simulink model "starship_sim"  (R2024b)
settings: Solver=VariableStepAuto  StartTime=0.0  StopTime=10  FixedStep=0.01
values from neighbouring files (symbols this model uses):
  A = [0   1   0   0   0   0    0    0    0    0 ... (first row only)    [LQR_FINAL.m]
  B = [0          0             0            0 ... (first row only)    [LQR_FINAL.m]
  C = eye(10)    [LQR_FINAL.m]
  m = 2.5    [LQR_FINAL.m]
undefined symbols (not defined in the file or in its folder): K, X, Y, Z
libraries: nesl_utility x31, sm_lib x28, sharedtransform x1
(part 1 of 2)
settings Model: Creator=gilli  LastModifiedBy=thurf
settings DebuggingCC: UnderSpecifiedDimensionMsg=error
settings SimscapeCC: SimscapeLogType=all

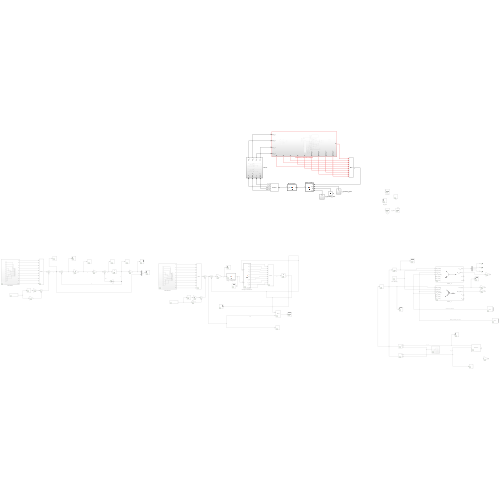
[thumbnail: Simulink's stored preview of the top-level diagram]
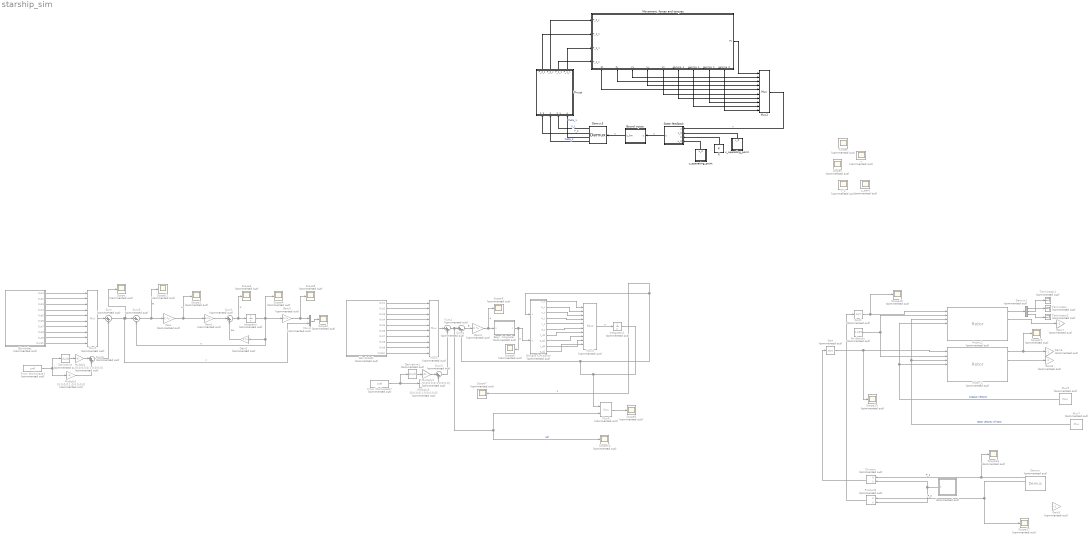
== system starship_sim ==
  " " : Subsystem  Commented=on
  Air density : Constant  Commented=on  Value=1.225
  Angles : Scope  Commented=on  NumInputPorts=2
  Begr. Insignaler : MATLAB Function  Commented=on  TreatAsAtomicUnit=on
  Bound inputs : MATLAB Function  TreatAsAtomicUnit=on
  Börvärdet : Subsystem  Commented=on
  Börvärdet1 : Subsystem  Commented=on
  Demux : Demux  Commented=on
      settings: DisplayOption=none
  Demux1 : Demux  Commented=on  Outputs=3
  Demux3 : Demux
      settings: DisplayOption=none
  Derivative : Derivative  Commented=on
  Derivative1 : Derivative  Commented=on
  Division : Product  Commented=on  Inputs=*/
  Forces : Scope  Commented=on  NumInputPorts=2
  From Workspace1 : FromWorkspace  Commented=on  VariableName=zref
  From Workspace2 : FromWorkspace  Commented=on  VariableName=zref
  Gain : Gain  Commented=on  Gain=K  Multiplication=Matrix(K*u)
  Gain1 : Gain  Commented=on  Gain=B  Multiplication=Matrix(K*u)
  Gain2 : Gain  Commented=on  Gain=A  Multiplication=Matrix(K*u)
  Gain3 : Gain  Commented=on  Gain=C  Multiplication=Matrix(K*u)
  Gain4 : Gain  Commented=on  Gain=K  Multiplication=Matrix(K*u)
  Gain{5..8} (4 alike) : Gain  Commented=on  Gain=-1
  Integrator : Integrator  Commented=on
  Integrator1 : Integrator  Commented=on
  K : Constant  Value=K
  "Movement, forces and torques" : Subsystem  VariantControl=VSS_MODE == 1
      settings: PortSchema="{\"entries\":[{\"content\":{\"sides\":[{\"content\":{\"connectorIds\":[\"In1\",\"In2\",\"In3\",\"In4\"]},\"type\":\"ConnectorPlacement.EquallySpacedRectSide\",\"uuid\":\"a8894a8f-a517-45d3-8d08-526e98f0b7fd\"},{\"content\":{\"connectorIds\":[\"Out1\"],\"side\":\"RIGHT\"},\"type\":\"ConnectorPlacement.EquallySpacedRectSide\",\"uuid\":\"ae51d042-9e2e-4067-8d07-01ed82c4b16d\"},{\"content\":{\"side\":\"TOP\"},\"type\":\"ConnectorPlacement.EquallySpacedRectSide\",\"uuid\":\"be1ac344-a561-48a5-8df5-808c22469c33\"},{\"content\":{\"connectorIds\":[\"Out2\",\"Out3\",\"Out4\",\"Out5\",\"Out6\",\"Out7\",\"Out8\",\"Out9\",\"Out10\"],\"side\":\"BOTTOM\"},\"type\":\"ConnectorPlacement.EquallySpacedRectSide\",\"uuid\":\"6ea89cb2-a822-4d68-9844-f5d3e0b45fc4\"}]},\"type\":\"ConnectorPlacement.EquallySpacedConnector\",\"uuid\":\"3addfc64-b65f-46cf-8b70-884cdc71d4e0\"}],\"packageUris\":[\"http://schema.mathworks.com/mf0/Connector/R2020b\"],\"version\":\"1.0\"}"
  Multiply : Gain  Commented=on  Gain=[0;0;0;0;0;1;0;0;0;0]
  Multiply1 : Gain  Commented=on  Gain=[0;0;0;0;1;0;0;0;0;0]
  Multiply2 : Gain  Commented=on  Gain=[0;0;0;0;0;1;0;0;0;0]
  Multiply3 : Gain  Commented=on  Gain=[0;0;0;0;1;0;0;0;0;0]
  Mux1 : Mux  Commented=on  Inputs=10
  Mux2 : Mux  Inputs=10
  Mux3 : Mux  Commented=on  Inputs=2
  Mux4 : Mux  Commented=on  Inputs=10
  Mux5 : Mux  Commented=on  Inputs=10
  Mux6 : Mux  Commented=on  Inputs=2
  Mux7 : Mux  Commented=on  Inputs=3
  Mux9 : Mux  Commented=on  Inputs=3
  Olinjära funktioner : MATLAB Function  Commented=on  TreatAsAtomicUnit=on
  Product2 : Product  Commented=on  Inputs=*/
  Rotor_1 : Rotor  Commented=on  modelMode=With flap effects  controlInput=on  CTCQMode=Compute using BEMT  Nb=3  CTout=on  radius=0.102  chord=0.098  cd0=0.03
  Rotor_2 : Rotor  Commented=on  modelMode=With flap effects  controlInput=on  CTCQMode=Compute using BEMT  Nb=3  CTout=on  radius=0.102  chord=0.098  cd0=0.03
  Scope{,1..11,15..19} (17 alike) : Scope  Commented=on
  Sqrt : Sqrt  Commented=on
  Sqrt1 : Sqrt  Commented=on
  State feedback : MATLAB Function  TreatAsAtomicUnit=on
  Sum{,1..3,6} (5 alike) : Sum  Commented=on  Inputs=|++
  Sum4 : Sum  Commented=on  Inputs=|+-
  Sum5 : Sum  Commented=on  Inputs=|+-
  Terminator : Terminator  Commented=on
  Terminator1 : Terminator  Commented=on
  Terminator2 : Terminator  Commented=on
  Thrust : Subsystem
  u_operating_point : Subsystem
  u_start : Scope  Commented=on
  x : Scope  Commented=on
  x_0 : Scope  Commented=on
  x_operating_point : Subsystem
  wires:
  Olinjära funktioner/1(v_x) -> Mux4/1
  Olinjära funktioner/2(a_x) -> Mux4/2
  Olinjära funktioner/3(v_y) -> Mux4/3
  Olinjära funktioner/4(a_y) -> Mux4/4
  Olinjära funktioner/5(v_z) -> Mux4/5
  Olinjära funktioner/7(v_g1) -> Mux4/7
  Olinjära funktioner/8(a_g1) -> Mux4/8
  Olinjära funktioner/9(v_g2) -> Mux4/9
  Olinjära funktioner/10(a_g2) -> Mux4/10
  Mux1/1 -> Sum/1
  Börvärdet/1(Out1) -> Mux1/1
  Börvärdet/2(Out2) -> Mux1/2
  Börvärdet/3(Out3) -> Mux1/3
  Börvärdet/4(Out4) -> Mux1/4
  Börvärdet/5(Out5) -> Mux1/5
  Börvärdet/6(Out6) -> Mux1/6
  Börvärdet/7(Out7) -> Mux1/7
  Börvärdet/8(Out8) -> Mux1/8
  Börvärdet/9(Out9) -> Mux1/9
  Börvärdet/10(Out10) -> Mux1/10
  Sum6/1 -> Sum/2
  From Workspace1/1 -> Derivative/1, Multiply1/1
  Multiply1/1 -> Sum6/2
  Multiply/1 -> Sum6/1
  Derivative/1 -> Multiply/1
  Gain1/1 -> Sum1/1
  Gain2/1 -> Sum1/2  "Ax"
  Sum1/1 -> Scope3/1, Integrator/1  "x'"
  Integrator/1 -> Sum5/2, Gain2/1, Gain3/1, Scope4/1  "x"
  Gain/1 -> Gain1/1, Scope1/1  "u"
  Gain3/1 -> Scope5/1, Mux3/1
  Mux3/1 -> Scope2/1
  Derivative1/1 -> Multiply2/1
  From Workspace2/1 -> Multiply3/1, Derivative1/1
  Multiply3/1 -> Sum3/2
  Börvärdet1/5(Out5) -> Mux5/5
  Börvärdet1/7(Out7) -> Mux5/7
  Börvärdet1/4(Out4) -> Mux5/4
  Börvärdet1/6(Out6) -> Mux5/6
  Börvärdet1/3(Out3) -> Mux5/3
  Börvärdet1/1(Out1) -> Mux5/1
  Börvärdet1/2(Out2) -> Mux5/2
  Börvärdet1/8(Out8) -> Mux5/8
  Börvärdet1/9(Out9) -> Mux5/9
  Börvärdet1/10(Out10) -> Mux5/10
  Mux5/1 -> Sum2/1
  Multiply2/1 -> Sum3/1
  Sum3/1 -> Sum2/2
  Gain4/1 -> Scope9/1, Begr. Insignaler/1(u)  "u"
  Begr. Insignaler/1(y) -> Scope6/1, Olinjära funktioner/2(u)  "u"
  Sum2/1 -> Scope10/1, Mux6/2, Sum4/1  "ref"
  Sum4/1 -> Gain4/1  "e"
  Mux6/1 -> Scope8/1
  Mux4/1 -> Integrator1/1  "x'"
  Olinjära funktioner/6(a_z) -> Mux4/6
  Sum/1 -> Mux3/2, Scope/1, Sum5/1  "r"
  Sum5/1 -> Scope11/1, Gain/1  "e"
  Integrator1/1 -> Mux6/1, Scope7/1, Olinjära funktioner/1(x), Sum4/2  "x"
  Mux7/1 -> Rotor_1/3, Rotor_2/3  "Body velocity of rotor"
  Mux9/1 -> Rotor_1/4, Rotor_2/4  "Angular velocity"
  Rotor_1/1 -> Scope15/1, Gain6/1
  Rotor_2/2 -> Gain7/1
  Demux/1 -> Scope16/1, Division/1  "F_1"
  Demux/2 -> Scope17/1, Product2/1  "F_2"
  Division/1 -> Sqrt/1
  Product2/1 -> Sqrt1/1
  Rotor_1/2 -> Gain8/1
  State feedback/1(u) -> Bound inputs/1(u)  "u"
  x_operating_point/1(x_0) -> State feedback/2(x_0)
  Air density/1 -> Rotor_1/2, Rotor_2/2
  Sqrt/1 -> Scope19/1, Rotor_1/1
  Sqrt1/1 -> Scope18/1, Rotor_2/1
  " "/1(" ") -> Division/2, Product2/2
  Rotor_2/1 -> Demux1/1
  Demux1/1 -> Terminator/1
  Demux1/3 -> Terminator2/1
  Demux1/2 -> Terminator1/1
  Mux2/1 -> State feedback/1(x)  "x"
  Demux3/1 -> Thrust/3(F_1)  "F_1"
  Demux3/2 -> Thrust/1(F_2)  "F_2"
  Demux3/3 -> Thrust/4(theta_1)  "theta_1"
  Demux3/4 -> Thrust/2(theta_2)  "theta_2"
  Thrust/4(F_1_x) -> "Movement, forces and torques"/3(F_1_x)
  Thrust/3(F_1_z) -> "Movement, forces and torques"/4(F_1_z)
  Thrust/2(F_2_y) -> "Movement, forces and torques"/1(F_2_y)
  Thrust/1(F_2_z) -> "Movement, forces and torques"/2(F_2_z)
  "Movement, forces and torques"/1(Px) -> Mux2/1
  "Movement, forces and torques"/4(Vx) -> Mux2/2
  "Movement, forces and torques"/3(Py) -> Mux2/3
  "Movement, forces and torques"/5(Vy) -> Mux2/4
  "Movement, forces and torques"/2(Pz) -> Mux2/5
  "Movement, forces and torques"/6(Vz) -> Mux2/6
  "Movement, forces and torques"/7(gamma_1) -> Mux2/7
  "Movement, forces and torques"/9(gamma_1') -> Mux2/8
  "Movement, forces and torques"/8(gamma_2) -> Mux2/9
  "Movement, forces and torques"/10(gamma_2') -> Mux2/10
  K/1 -> State feedback/3(K)
  u_operating_point/1(u_0) -> State feedback/4(u_0)
  Bound inputs/1(u_lim) -> Demux3/1  "u"

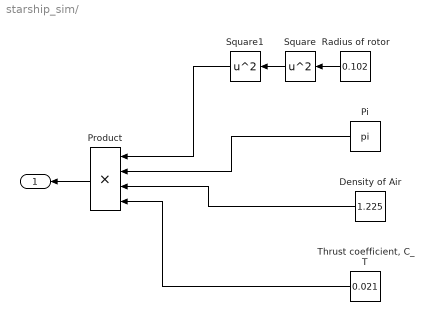
== system starship_sim/  ==
  Density of Air : Constant  Value=1.225
  Pi : Constant  Value=pi  OutDataTypeStr=Inherit: Inherit via back propagation
  Product : Product  Inputs=4
  Radius of rotor : Constant  Value=0.102
  Square : Math  Operator=square
  Square1 : Math  Operator=square
  "Thrust coefficient, C_T" : Constant  Value=0.021
  " " : Outport
  wires:
  Density of Air/1 -> Product/3
  Product/1 -> " "/1
  Pi/1 -> Product/2
  "Thrust coefficient, C_T"/1 -> Product/4
  Square/1 -> Square1/1
  Radius of rotor/1 -> Square/1
  Square1/1 -> Product/1

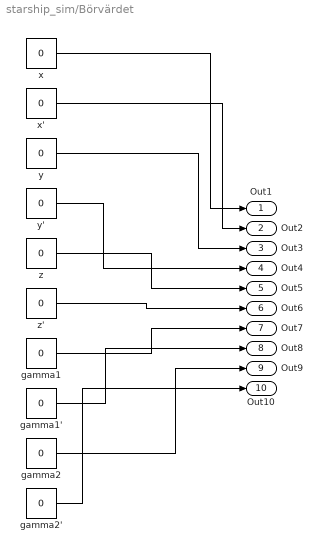
== system starship_sim/Börvärdet ==
  gamma1 : Constant  Value=0
  gamma1' : Constant  Value=0
  gamma2 : Constant  Value=0
  gamma2' : Constant  Value=0
  x : Constant  Value=0
  x' : Constant  Value=0
  y : Constant  Value=0
  y' : Constant  Value=0
  z : Constant  Value=0
  z' : Constant  Value=0
  Out1 : Outport
  Out2 : Outport  Port=2
  Out3 : Outport  Port=3
  Out4 : Outport  Port=4
  Out5 : Outport  Port=5
  Out6 : Outport  Port=6
  Out7 : Outport  Port=7
  Out8 : Outport  Port=8
  Out9 : Outport  Port=9
  Out10 : Outport  Port=10
  wires:
  gamma1/1 -> Out7/1
  gamma1'/1 -> Out8/1
  y/1 -> Out3/1
  gamma2/1 -> Out9/1
  x/1 -> Out1/1
  gamma2'/1 -> Out10/1
  y'/1 -> Out4/1
  z/1 -> Out5/1
  z'/1 -> Out6/1
  x'/1 -> Out2/1

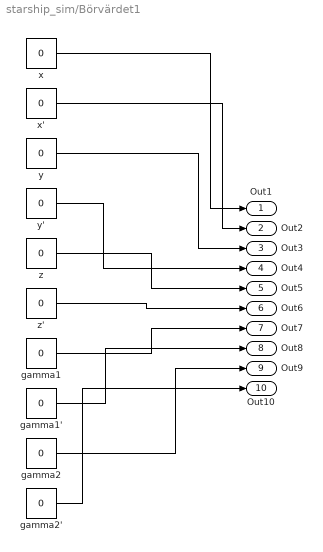
== system starship_sim/Börvärdet1 ==
  gamma1 : Constant  Value=0
  gamma1' : Constant  Value=0
  gamma2 : Constant  Value=0
  gamma2' : Constant  Value=0
  x : Constant  Value=0
  x' : Constant  Value=0
  y : Constant  Value=0
  y' : Constant  Value=0
  z : Constant  Value=0
  z' : Constant  Value=0
  Out1 : Outport
  Out2 : Outport  Port=2
  Out3 : Outport  Port=3
  Out4 : Outport  Port=4
  Out5 : Outport  Port=5
  Out6 : Outport  Port=6
  Out7 : Outport  Port=7
  Out8 : Outport  Port=8
  Out9 : Outport  Port=9
  Out10 : Outport  Port=10
  wires:
  gamma1/1 -> Out7/1
  gamma1'/1 -> Out8/1
  y/1 -> Out3/1
  gamma2/1 -> Out9/1
  x/1 -> Out1/1
  gamma2'/1 -> Out10/1
  y'/1 -> Out4/1
  z/1 -> Out5/1
  z'/1 -> Out6/1
  x'/1 -> Out2/1

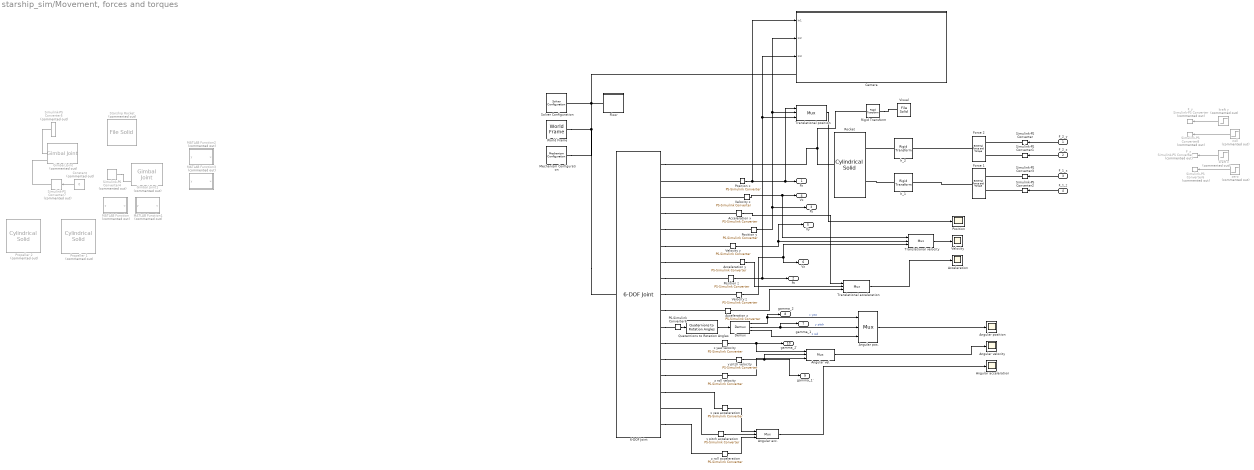
== system starship_sim/Movement, forces and torques ==
  F_2_y : Inport
  F_2_z : Inport  Port=2
  F_1_x : Inport  Port=3
  F_1_z : Inport  Port=4
  6-DOF Joint : sm_lib/Joints/6-DOF Joint  JointMode=Normal  CompositeWrenchDir=FollowerOnBase  CompositeWrenchFrame=BaseFrame  SenseConstraintForce=off  SenseConstraintTorque=off  SenseTotalForce=off  SenseTotalTorque=off  PxPositionTargetSpecify=off  PxPositionTargetPriority=High  PxPositionTargetValue=0  PxPositionTargetValueUnits=m  PxVelocityTargetSpecify=off  PxVelocityTargetPriority=High  PxVelocityTargetValue=0  PxVelocityTargetValueUnits=m/s  PxEquilibriumPosition=0  PxEquilibriumPositionUnits=m  PxSpringStiffness=0  PxSpringStiffnessUnits=N/m  PxDampingCoefficient=0  PxDampingCoefficientUnits=N/(m/s)  PxLowerLimitSpecify=off  PxLowerLimitBound=-1  PxLowerLimitBoundUnits=m  PxLowerLimitStiffness=1e6  PxLowerLimitStiffnessUnits=N/m  PxLowerLimitDamping=1e3  PxLowerLimitDampingUnits=N/(m/s)  PxLowerLimitTransitionRegionWidth=1e-4  PxLowerLimitTransitionRegionWidthUnits=m  PxUpperLimitSpecify=off  PxUpperLimitBound=1  PxUpperLimitBoundUnits=m  PxUpperLimitStiffness=1e6  PxUpperLimitStiffnessUnits=N/m  PxUpperLimitDamping=1e3  PxUpperLimitDampingUnits=N/(m/s)  PxUpperLimitTransitionRegionWidth=1e-4  PxUpperLimitTransitionRegionWidthUnits=m  PxTorqueActuationMode=NoTorque  PxMotionActuationMode=ComputedMotion  PxSensePosition=on  PxSenseVelocity=on  PxSenseAcceleration=on  PxSenseTorqueForce=off  PxSenseLowerLimitTorqueForce=off  PxSenseUpperLimitTorqueForce=off  PyPositionTargetSpecify=off  PyPositionTargetPriority=High  PyPositionTargetValue=0  PyPositionTargetValueUnits=m  PyVelocityTargetSpecify=off  PyVelocityTargetPriority=High  PyVelocityTargetValue=0  PyVelocityTargetValueUnits=m/s  PyEquilibriumPosition=0  PyEquilibriumPositionUnits=m  PySpringStiffness=0  PySpringStiffnessUnits=N/m  PyDampingCoefficient=0  PyDampingCoefficientUnits=N/(m/s)  PyLowerLimitSpecify=off  PyLowerLimitBound=-1  PyLowerLimitBoundUnits=m  PyLowerLimitStiffness=1e6  PyLowerLimitStiffnessUnits=N/m  PyLowerLimitDamping=1e3  PyLowerLimitDampingUnits=N/(m/s)  PyLowerLimitTransitionRegionWidth=1e-4  PyLowerLimitTransitionRegionWidthUnits=m  PyUpperLimitSpecify=off  PyUpperLimitBound=1  PyUpperLimitBoundUnits=m  PyUpperLimitStiffness=1e6  PyUpperLimitStiffnessUnits=N/m  PyUpperLimitDamping=1e3  PyUpperLimitDampingUnits=N/(m/s)  PyUpperLimitTransitionRegionWidth=1e-4  PyUpperLimitTransitionRegionWidthUnits=m  PyTorqueActuationMode=NoTorque  PyMotionActuationMode=ComputedMotion  PySensePosition=on  PySenseVelocity=on  PySenseAcceleration=on  PySenseTorqueForce=off  PySenseLowerLimitTorqueForce=off  PySenseUpperLimitTorqueForce=off  PzPositionTargetSpecify=off  PzPositionTargetPriority=High  PzPositionTargetValue=0  PzPositionTargetValueUnits=m  PzVelocityTargetSpecify=off  PzVelocityTargetPriority=High  PzVelocityTargetValue=0  PzVelocityTargetValueUnits=m/s  PzEquilibriumPosition=0  PzEquilibriumPositionUnits=m  PzSpringStiffness=0  PzSpringStiffnessUnits=N/m  PzDampingCoefficient=0  PzDampingCoefficientUnits=N/(m/s)  PzLowerLimitSpecify=off  PzLowerLimitBound=0  PzLowerLimitBoundUnits=m  PzLowerLimitStiffness=100  PzLowerLimitStiffnessUnits=N/m  PzLowerLimitDamping=1e3  PzLowerLimitDampingUnits=N/(m/s)  PzLowerLimitTransitionRegionWidth=1e-4  PzLowerLimitTransitionRegionWidthUnits=m  PzUpperLimitSpecify=off  PzUpperLimitBound=10  PzUpperLimitBoundUnits=m  PzUpperLimitStiffness=1e6  PzUpperLimitStiffnessUnits=N/m  PzUpperLimitDamping=1e3  PzUpperLimitDampingUnits=N/(m/s)  PzUpperLimitTransitionRegionWidth=1e-4  PzUpperLimitTransitionRegionWidthUnits=m  PzTorqueActuationMode=NoTorque  PzMotionActuationMode=ComputedMotion  PzSensePosition=on  PzSenseVelocity=on  PzSenseAcceleration=on  PzSenseTorqueForce=off  PzSenseLowerLimitTorqueForce=off  PzSenseUpperLimitTorqueForce=off  SphPositionTargetSpecify=off  SphPositionTargetPriority=High  SphPositionTargetRotationMethod=AlignedAxes  SphPositionTargetFollAlignAxisA=+X  SphPositionTargetBaseAlignAxisA=+Y  SphPositionTargetFollAlignAxisB=+Y  SphPositionTargetBaseAlignAxisB=+Z  SphPositionTargetRotationStandardAxis=+Z  SphPositionTargetRotationAngle=0.0  SphPositionTargetRotationAngleUnits=deg  SphPositionTargetRotationArbitraryAxis=[0 0 1]  SphPositionTargetRotationSequenceAxes=FollowerAxes  SphPositionTargetRotationSequence=XYX  SphPositionTargetRotationSequenceAngles=[0 0 0]  SphPositionTargetRotationSequenceAnglesUnits=deg  SphPositionTargetRotationMatrix=[1 0 0; 0 1 0; 0 0 1]  SphPositionTargetQuaternion=[1 0 0 0]  SphVelocityTargetSpecify=off  SphVelocityTargetPriority=High  SphVelocityTargetValue=[0 0 0]  SphVelocityTargetValueUnits=deg/s  SphVelocityTargetInFollowerFrame=on  SphEqPosRotationMethod=None  SphEqPosFollAlignAxisA=+X  SphEqPosBaseAlignAxisA=+Y  SphEqPosFollAlignAxisB=+Y  SphEqPosBaseAlignAxisB=+Z  SphEqPosRotationStandardAxis=+Z  SphEqPosRotationAngle=0.0  SphEqPosRotationAngleUnits=deg  SphEqPosRotationArbitraryAxis=[0 0 1]  SphEqPosRotationSequenceAxes=FollowerAxes  SphEqPosRotationSequence=XYX  SphEqPosRotationSequenceAngles=[0 0 0]  SphEqPosRotationSequenceAnglesUnits=deg  SphEqPosRotationMatrix=[1 0 0; 0 1 0; 0 0 1]  SphEqPosQuaternion=[1 0 0 0]  SphSpringStiffness=0  SphSpringStiffnessUnits=N*m/deg  SphDampingCoefficient=0  SphDampingCoefficientUnits=N*m/(deg/s)  SphLowerLimitSpecify=off  SphLowerLimitBound=15  SphLowerLimitBoundUnits=deg  SphLowerLimitStiffness=1e4  SphLowerLimitStiffnessUnits=N*m/deg  SphLowerLimitDamping=10  SphLowerLimitDampingUnits=N*m/(deg/s)  SphLowerLimitTransitionRegionWidth=0.1  SphLowerLimitTransitionRegionWidthUnits=deg  SphUpperLimitSpecify=off  SphUpperLimitBound=45  SphUpperLimitBoundUnits=deg  SphUpperLimitStiffness=1e4  SphUpperLimitStiffnessUnits=N*m/deg  SphUpperLimitDamping=10  SphUpperLimitDampingUnits=N*m/(deg/s)  SphUpperLimitTransitionRegionWidth=0.1  SphUpperLimitTransitionRegionWidthUnits=deg  SphTorqueActuationMode=InputTorque  SphActuateTorqueX=off  SphActuateTorqueY=off  SphActuateTorqueZ=off  SphActuateTorque=off  SphActuationFrame=BaseFrame  SphSensePosition=on  SphSenseVelocityX=on  SphSenseVelocityY=on  SphSenseVelocityZ=on  SphSenseVelocity=off  SphSenseAccelerationX=on  SphSenseAccelerationY=on  SphSenseAccelerationZ=on  SphSenseAcceleration=off  SphSenseLowerLimitTorqueMag=off  SphSenseUpperLimitTorqueMag=off  SphSensingFrame=BaseFrame
  Acceleration : Scope
  Acceleration x : nesl_utility/PS-Simulink Converter  PhysicalDomain=network_engine_domain  SubClassName=ps_output  LeftPortType=input  RightPortType=output  PseudoPeriodic=off  Frequencies=[]  VectorFormat=1-D array  Unit=inherit  AffineConversion=off
  Acceleration y : nesl_utility/PS-Simulink Converter  PhysicalDomain=network_engine_domain  SubClassName=ps_output  LeftPortType=input  RightPortType=output  PseudoPeriodic=off  Frequencies=[]  VectorFormat=1-D array  Unit=inherit  AffineConversion=off
  Acceleration z : nesl_utility/PS-Simulink Converter  PhysicalDomain=network_engine_domain  SubClassName=ps_output  LeftPortType=input  RightPortType=output  PseudoPeriodic=off  Frequencies=[]  VectorFormat=1-D array  Unit=inherit  AffineConversion=off
  Angular acc. : Mux  Inputs=3
  Angular acceleration : Scope
  Angular pos. : Mux  Inputs=3
  Angular position : Scope
  Angular vel. : Mux  Inputs=3
  Angular velocity : Scope
  Camera : Subsystem
  Constant : Constant  Commented=on  Value=0
  Demux : Demux  Outputs=3
      settings: DisplayOption=none
  F_x : nesl_utility/Simulink-PS Converter  Commented=on  PhysicalDomain=network_engine_domain  SubClassName=ps_input  LeftPortType=input  RightPortType=output  PseudoPeriodic=off  Frequencies=[]  NoiseDistribution=none  NoiseParameters=[]  Unit=1  AffineConversion=off  FilteringAndDerivatives=provide  SimscapeFilterOrder=1  InputFilterTimeConstant=0.001  UdotUserProvided=0
  F_y : nesl_utility/Simulink-PS Converter  Commented=on  PhysicalDomain=network_engine_domain  SubClassName=ps_input  LeftPortType=input  RightPortType=output  PseudoPeriodic=off  Frequencies=[]  NoiseDistribution=none  NoiseParameters=[]  Unit=1  AffineConversion=off  FilteringAndDerivatives=provide  SimscapeFilterOrder=1  InputFilterTimeConstant=0.001  UdotUserProvided=0
  Floor : Subsystem
  Force 1 : sm_lib/Forces and Torques/External Force and Torque  EnableForceX=on  EnableForceY=off  EnableForceZ=on  EnableForce=off  ForceResolutionFrame=AttachedFrame  EnableTorqueX=off  EnableTorqueY=off  EnableTorqueZ=off  EnableTorque=off  TorqueResolutionFrame=AttachedFrame
  Force 2 : sm_lib/Forces and Torques/External Force and Torque  EnableForceX=off  EnableForceY=on  EnableForceZ=on  EnableForce=off  ForceResolutionFrame=AttachedFrame  EnableTorqueX=off  EnableTorqueY=off  EnableTorqueZ=off  EnableTorque=off  TorqueResolutionFrame=AttachedFrame
  Gimbal Joint : sm_lib/Joints/Gimbal Joint  Commented=on  JointMode=Normal  CompositeWrenchDir=FollowerOnBase  CompositeWrenchFrame=BaseFrame  SenseConstraintForce=off  SenseConstraintTorque=off  SenseTotalForce=off  SenseTotalTorque=off  RxPositionTargetSpecify=off  RxPositionTargetPriority=High  RxPositionTargetValue=30  RxPositionTargetValueUnits=deg  RxVelocityTargetSpecify=off  RxVelocityTargetPriority=High  RxVelocityTargetValue=0  RxVelocityTargetValueUnits=deg/s  RxEquilibriumPosition=0  RxEquilibriumPositionUnits=deg  RxSpringStiffness=0  RxSpringStiffnessUnits=N*m/deg  RxDampingCoefficient=0  RxDampingCoefficientUnits=N*m/(deg/s)  RxLowerLimitSpecify=on  RxLowerLimitBound=-45  RxLowerLimitBoundUnits=deg  RxLowerLimitStiffness=1e4  RxLowerLimitStiffnessUnits=N*m/deg  RxLowerLimitDamping=10  RxLowerLimitDampingUnits=N*m/(deg/s)  RxLowerLimitTransitionRegionWidth=0.1  RxLowerLimitTransitionRegionWidthUnits=deg  RxUpperLimitSpecify=on  RxUpperLimitBound=45  RxUpperLimitBoundUnits=deg  RxUpperLimitStiffness=1e4  RxUpperLimitStiffnessUnits=N*m/deg  RxUpperLimitDamping=10  RxUpperLimitDampingUnits=N*m/(deg/s)  RxUpperLimitTransitionRegionWidth=0.1  RxUpperLimitTransitionRegionWidthUnits=deg  RxTorqueActuationMode=ComputedTorque  RxMotionActuationMode=InputMotion  RxSensePosition=off  RxSenseVelocity=off  RxSenseAcceleration=off  RxSenseTorqueForce=off  RxSenseLowerLimitTorqueForce=off  RxSenseUpperLimitTorqueForce=off  RyPositionTargetSpecify=off  RyPositionTargetPriority=High  RyPositionTargetValue=0  RyPositionTargetValueUnits=deg  RyVelocityTargetSpecify=off  RyVelocityTargetPriority=High  RyVelocityTargetValue=0  RyVelocityTargetValueUnits=deg/s  RyEquilibriumPosition=0  RyEquilibriumPositionUnits=deg  RySpringStiffness=0  RySpringStiffnessUnits=N*m/deg  RyDampingCoefficient=0  RyDampingCoefficientUnits=N*m/(deg/s)  RyLowerLimitSpecify=off  RyLowerLimitBound=-90  RyLowerLimitBoundUnits=deg  RyLowerLimitStiffness=1e4  RyLowerLimitStiffnessUnits=N*m/deg  RyLowerLimitDamping=10  RyLowerLimitDampingUnits=N*m/(deg/s)  RyLowerLimitTransitionRegionWidth=0.1  RyLowerLimitTransitionRegionWidthUnits=deg  RyUpperLimitSpecify=off  RyUpperLimitBound=90  RyUpperLimitBoundUnits=deg  RyUpperLimitStiffness=1e4  RyUpperLimitStiffnessUnits=N*m/deg  RyUpperLimitDamping=10  RyUpperLimitDampingUnits=N*m/(deg/s)  RyUpperLimitTransitionRegionWidth=0.1  RyUpperLimitTransitionRegionWidthUnits=deg  RyTorqueActuationMode=ComputedTorque  RyMotionActuationMode=InputMotion  RySensePosition=off  RySenseVelocity=off  RySenseAcceleration=off  RySenseTorqueForce=off  RySenseLowerLimitTorqueForce=off  RySenseUpperLimitTorqueForce=off  RzPositionTargetSpecify=off  RzPositionTargetPriority=High  RzPositionTargetValue=0  RzPositionTargetValueUnits=deg  RzVelocityTargetSpecify=off  RzVelocityTargetPriority=High  RzVelocityTargetValue=0  RzVelocityTargetValueUnits=deg/s  RzEquilibriumPosition=0  RzEquilibriumPositionUnits=deg  RzSpringStiffness=0  RzSpringStiffnessUnits=N*m/deg  RzDampingCoefficient=0  RzDampingCoefficientUnits=N*m/(deg/s)  RzLowerLimitSpecify=off  RzLowerLimitBound=-90  RzLowerLimitBoundUnits=deg  RzLowerLimitStiffness=1e4  RzLowerLimitStiffnessUnits=N*m/deg  RzLowerLimitDamping=10  RzLowerLimitDampingUnits=N*m/(deg/s)  RzLowerLimitTransitionRegionWidth=0.1  RzLowerLimitTransitionRegionWidthUnits=deg  RzUpperLimitSpecify=off  RzUpperLimitBound=90  RzUpperLimitBoundUnits=deg  RzUpperLimitStiffness=1e4  RzUpperLimitStiffnessUnits=N*m/deg  RzUpperLimitDamping=10  RzUpperLimitDampingUnits=N*m/(deg/s)  RzUpperLimitTransitionRegionWidth=0.1  RzUpperLimitTransitionRegionWidthUnits=deg  RzTorqueActuationMode=NoTorque  RzMotionActuationMode=ComputedMotion  RzSensePosition=off  RzSenseVelocity=off  RzSenseAcceleration=off  RzSenseTorqueForce=off  RzSenseLowerLimitTorqueForce=off  RzSenseUpperLimitTorqueForce=off
  Gimbal Joint1 : sm_lib/Joints/Gimbal Joint  Commented=on  JointMode=Normal  CompositeWrenchDir=FollowerOnBase  CompositeWrenchFrame=BaseFrame  SenseConstraintForce=off  SenseConstraintTorque=off  SenseTotalForce=off  SenseTotalTorque=off  RxPositionTargetSpecify=off  RxPositionTargetPriority=High  RxPositionTargetValue=30  RxPositionTargetValueUnits=deg  RxVelocityTargetSpecify=off  RxVelocityTargetPriority=High  RxVelocityTargetValue=0  RxVelocityTargetValueUnits=deg/s  RxEquilibriumPosition=0  RxEquilibriumPositionUnits=deg  RxSpringStiffness=0  RxSpringStiffnessUnits=N*m/deg  RxDampingCoefficient=0  RxDampingCoefficientUnits=N*m/(deg/s)  RxLowerLimitSpecify=off  RxLowerLimitBound=-90  RxLowerLimitBoundUnits=deg  RxLowerLimitStiffness=1e4  RxLowerLimitStiffnessUnits=N*m/deg  RxLowerLimitDamping=10  RxLowerLimitDampingUnits=N*m/(deg/s)  RxLowerLimitTransitionRegionWidth=0.1  RxLowerLimitTransitionRegionWidthUnits=deg  RxUpperLimitSpecify=off  RxUpperLimitBound=90  RxUpperLimitBoundUnits=deg  RxUpperLimitStiffness=1e4  RxUpperLimitStiffnessUnits=N*m/deg  RxUpperLimitDamping=10  RxUpperLimitDampingUnits=N*m/(deg/s)  RxUpperLimitTransitionRegionWidth=0.1  RxUpperLimitTransitionRegionWidthUnits=deg  RxTorqueActuationMode=ComputedTorque  RxMotionActuationMode=InputMotion  RxSensePosition=off  RxSenseVelocity=off  RxSenseAcceleration=off  RxSenseTorqueForce=off  RxSenseLowerLimitTorqueForce=off  RxSenseUpperLimitTorqueForce=off  RyPositionTargetSpecify=off  RyPositionTargetPriority=High  RyPositionTargetValue=0  RyPositionTargetValueUnits=deg  RyVelocityTargetSpecify=off  RyVelocityTargetPriority=High  RyVelocityTargetValue=0  RyVelocityTargetValueUnits=deg/s  RyEquilibriumPosition=0  RyEquilibriumPositionUnits=deg  RySpringStiffness=0  RySpringStiffnessUnits=N*m/deg  RyDampingCoefficient=0  RyDampingCoefficientUnits=N*m/(deg/s)  RyLowerLimitSpecify=on  RyLowerLimitBound=-45  RyLowerLimitBoundUnits=deg  RyLowerLimitStiffness=1e4  RyLowerLimitStiffnessUnits=N*m/deg  RyLowerLimitDamping=10  RyLowerLimitDampingUnits=N*m/(deg/s)  RyLowerLimitTransitionRegionWidth=0.1  RyLowerLimitTransitionRegionWidthUnits=deg  RyUpperLimitSpecify=on  RyUpperLimitBound=45  RyUpperLimitBoundUnits=deg  RyUpperLimitStiffness=1e4  RyUpperLimitStiffnessUnits=N*m/deg  RyUpperLimitDamping=10  RyUpperLimitDampingUnits=N*m/(deg/s)  RyUpperLimitTransitionRegionWidth=0.1  RyUpperLimitTransitionRegionWidthUnits=deg  RyTorqueActuationMode=ComputedTorque  RyMotionActuationMode=InputMotion  RySensePosition=off  RySenseVelocity=off  RySenseAcceleration=off  RySenseTorqueForce=off  RySenseLowerLimitTorqueForce=off  RySenseUpperLimitTorqueForce=off  RzPositionTargetSpecify=off  RzPositionTargetPriority=High  RzPositionTargetValue=0  RzPositionTargetValueUnits=deg  RzVelocityTargetSpecify=off  RzVelocityTargetPriority=High  RzVelocityTargetValue=0  RzVelocityTargetValueUnits=deg/s  RzEquilibriumPosition=0  RzEquilibriumPositionUnits=deg  RzSpringStiffness=0  RzSpringStiffnessUnits=N*m/deg  RzDampingCoefficient=0  RzDampingCoefficientUnits=N*m/(deg/s)  RzLowerLimitSpecify=off  RzLowerLimitBound=-90  RzLowerLimitBoundUnits=deg  RzLowerLimitStiffness=1e4  RzLowerLimitStiffnessUnits=N*m/deg  RzLowerLimitDamping=10  RzLowerLimitDampingUnits=N*m/(deg/s)  RzLowerLimitTransitionRegionWidth=0.1  RzLowerLimitTransitionRegionWidthUnits=deg  RzUpperLimitSpecify=off  RzUpperLimitBound=90  RzUpperLimitBoundUnits=deg  RzUpperLimitStiffness=1e4  RzUpperLimitStiffnessUnits=N*m/deg  RzUpperLimitDamping=10  RzUpperLimitDampingUnits=N*m/(deg/s)  RzUpperLimitTransitionRegionWidth=0.1  RzUpperLimitTransitionRegionWidthUnits=deg  RzTorqueActuationMode=NoTorque  RzMotionActuationMode=ComputedMotion  RzSensePosition=off  RzSenseVelocity=off  RzSenseAcceleration=off  RzSenseTorqueForce=off  RzSenseLowerLimitTorqueForce=off  RzSenseUpperLimitTorqueForce=off
  MATLAB Function : MATLAB Function  Commented=on  TreatAsAtomicUnit=on
  MATLAB Function1 : MATLAB Function  Commented=on  TreatAsAtomicUnit=on
  MATLAB Function2 : MATLAB Function  Commented=on  TreatAsAtomicUnit=on
  MATLAB Function3 : MATLAB Function  Commented=on  TreatAsAtomicUnit=on
  Mechanism Configuration : sm_lib/Utilities/Mechanism Configuration  UniformGravity=Constant  GravityVector=[0 0 -9.82]  GravityVectorUnits=m/s^2  LinearizationDelta=0.001  JointModeTransitionNonlinearIterations=2
  PS-Simulink Converter6 : nesl_utility/PS-Simulink Converter  PhysicalDomain=network_engine_domain  SubClassName=ps_output  LeftPortType=input  RightPortType=output  PseudoPeriodic=off  Frequencies=[]  VectorFormat=1-D array  Unit=inherit  AffineConversion=off
  Position : Scope
  Position x : nesl_utility/PS-Simulink Converter  PhysicalDomain=network_engine_domain  SubClassName=ps_output  LeftPortType=input  RightPortType=output  PseudoPeriodic=off  Frequencies=[]  VectorFormat=1-D array  Unit=inherit  AffineConversion=off
  Position y : nesl_utility/PS-Simulink Converter  PhysicalDomain=network_engine_domain  SubClassName=ps_output  LeftPortType=input  RightPortType=output  PseudoPeriodic=off  Frequencies=[]  VectorFormat=1-D array  Unit=inherit  AffineConversion=off
  Position z : nesl_utility/PS-Simulink Converter  PhysicalDomain=network_engine_domain  SubClassName=ps_output  LeftPortType=input  RightPortType=output  PseudoPeriodic=off  Frequencies=[]  VectorFormat=1-D array  Unit=inherit  AffineConversion=off
  Propeller 1 : sm_lib/Body Elements/Cylindrical Solid  Commented=on  CylinderRadius=0.102  CylinderRadiusUnits=m  CylinderLength=1  CylinderLengthUnits=cm  ExportEntireGeometry=off  InertiaType=Custom  BasedOnType=Density  Density=1000  DensityUnits=kg/m^3  Mass=10.3  MassUnits=g  CenterOfMass=[0 0 0]  CenterOfMassUnits=m  MomentsOfInertia=[50 0.1 0.1]  MomentsOfInertiaUnits=kg*m^2  ProductsOfInertia=[0 0 0]  ProductsOfInertiaUnits=kg*m^2  GraphicType=FromGeometry  MarkerShape=Sphere  MarkerSize=10  GraphicVisPropType=SimpleVisualProperties  GraphicDiffuseColor=[0.6 0.3 0.5]  GraphicOpacity=1  GraphicSpecularColor=[0.5 0.5 0.5 1.0]  GraphicAmbientColor=[0.15 0.15 0.15 1.0]  GraphicEmissiveColor=[0.0 0.0 0.0 1.0]  GraphicShininess=75  DoExposeReferenceFrame=on  SerializedFrames=<Frames><Frame><Id>Frame1</Id><Value><Name>Midpoint</Name><Origin><Source>ReferenceFrame</Source><FeatureName></FeatureName></Origin><PrimaryAxis><DefinedDirection>+Z</DefinedDirection><Source>ReferenceFrame</Source><SourceDirection>+Z</SourceDirection><FeatureName></FeatureName></PrimaryAxis><SecondaryAxis><DefinedDirection>+X</DefinedDirection><Source>ReferenceFrame</Source><SourceDirection>+X</SourceDirection><FeatureName></FeatureName></SecondaryAxis></Value></Frame></Frames>
  Propeller 2 : sm_lib/Body Elements/Cylindrical Solid  Commented=on  CylinderRadius=0.102  CylinderRadiusUnits=m  CylinderLength=1  CylinderLengthUnits=cm  ExportEntireGeometry=off  InertiaType=Custom  BasedOnType=Density  Density=1000  DensityUnits=kg/m^3  Mass=10.3  MassUnits=g  CenterOfMass=[0 0 0]  CenterOfMassUnits=m  MomentsOfInertia=[0.1 50 0.1]  MomentsOfInertiaUnits=kg*m^2  ProductsOfInertia=[0 0 0]  ProductsOfInertiaUnits=kg*m^2  GraphicType=FromGeometry  MarkerShape=Sphere  MarkerSize=10  GraphicVisPropType=SimpleVisualProperties  GraphicDiffuseColor=[0.3 0.6 0.5]  GraphicOpacity=1  GraphicSpecularColor=[0.5 0.5 0.5 1.0]  GraphicAmbientColor=[0.15 0.15 0.15 1.0]  GraphicEmissiveColor=[0.0 0.0 0.0 1.0]  GraphicShininess=75  DoExposeReferenceFrame=on  SerializedFrames=<Frames><Frame><Id>Frame1</Id><Value><Name>Midpoint</Name><Origin><Source>ReferenceFrame</Source><FeatureName></FeatureName></Origin><PrimaryAxis><DefinedDirection>+Z</DefinedDirection><Source>ReferenceFrame</Source><SourceDirection>+Z</SourceDirection><FeatureName></FeatureName></PrimaryAxis><SecondaryAxis><DefinedDirection>+X</DefinedDirection><Source>ReferenceFrame</Source><SourceDirection>+X</SourceDirection><FeatureName></FeatureName></SecondaryAxis></Value></Frame></Frames>
  Quaternions to Rotation Angles : sharedtransform/Quaternions to Rotation Angles  rotationOrder=XYZ  aMode=aMode
  Rigid Transform : sm_lib/Frames and Transforms/Rigid Transform  RotationMethod=None  FollAlignAxisA=+X  BaseAlignAxisA=+Y  FollAlignAxisB=+Y  BaseAlignAxisB=+Z  RotationStandardAxis=+Z  RotationAngle=0  RotationAngleUnits=deg  RotationArbitraryAxis=[0 0 1]  RotationSequenceAxes=FollowerAxes  RotationSequence=XYX  RotationSequenceAngles=[0 0 0]  RotationSequenceAnglesUnits=deg  RotationMatrix=[1 0 0;0 1 0;0 0 1]  Quaternion=[1 0 0 0]  TranslationMethod=Cartesian  TranslationCartesianOffset=[0 0 -1143.2]  TranslationCartesianOffsetUnits=mm  TranslationStandardAxis=+Z  TranslationStandardOffset=0  TranslationStandardOffsetUnits=m  TranslationROffset=0  TranslationROffsetUnits=m  TranslationThetaOffset=0  TranslationThetaOffsetUnits=deg  TranslationZOffset=0  TranslationZOffsetUnits=m
  Rocket : sm_lib/Body Elements/Cylindrical Solid  CylinderRadius=137.5  CylinderRadiusUnits=mm  CylinderLength=1000  CylinderLengthUnits=mm  ExportEntireGeometry=off  InertiaType=Custom  BasedOnType=Density  Density=1000  DensityUnits=kg/m^3  Mass=3  MassUnits=kg  CenterOfMass=[66 38 34]  CenterOfMassUnits=mm  MomentsOfInertia=[0.215 0.226 0.042]  MomentsOfInertiaUnits=kg*m^2  ProductsOfInertia=[0 0 0]  ProductsOfInertiaUnits=kg*m^2  GraphicType=FromGeometry  MarkerShape=Sphere  MarkerSize=10  GraphicVisPropType=SimpleVisualProperties  GraphicDiffuseColor=[0.851 0.3255 0.09804]  GraphicOpacity=0  GraphicSpecularColor=[0.5 0.5 0.5 1.0]  GraphicAmbientColor=[0.15 0.15 0.15 1.0]  GraphicEmissiveColor=[0.0 0.0 0.0 1.0]  GraphicShininess=75  DoExposeReferenceFrame=on  SerializedFrames=<Frames><Frame><Id>Frame1</Id><Value><Name>Upper motor</Name><Origin><Source>ReferenceFrame</Source><FeatureName></FeatureName></Origin><PrimaryAxis><DefinedDirection>+Z</DefinedDirection><Source>ReferenceFrame</Source><SourceDirection>+Z</SourceDirection><FeatureName></FeatureName></PrimaryAxis><SecondaryAxis><DefinedDirection>+X</DefinedDirection><Source>ReferenceFrame</Source><SourceDirection>+X</SourceDirection><FeatureName></FeatureName></SecondaryAxis></Value></Frame><Frame><Id>Frame2</Id><Value><Name>Lower motor</Name><Origin><Source>ReferenceFrame</Source><FeatureName></FeatureName></Origin><PrimaryAxis><DefinedDirection>+Z</DefinedDirection><Source>ReferenceFrame</Source><SourceDirection>+Z</SourceDirection><FeatureName></FeatureName></PrimaryAxis><SecondaryAxis><DefinedDirection>+X</DefinedDirection><Source>ReferenceFrame</Source><SourceDirection>+X</SourceDirection><FeatureName></FeatureName></SecondaryAxis></Value></Frame></Frames>
  Simulink-PS Converter{,1..3} (4 alike) : nesl_utility/Simulink-PS Converter  PhysicalDomain=network_engine_domain  SubClassName=ps_input  LeftPortType=input  RightPortType=output  PseudoPeriodic=off  Frequencies=[]  NoiseDistribution=none  NoiseParameters=[]  Unit=1  AffineConversion=off  FilteringAndDerivatives=provide  SimscapeFilterOrder=1  InputFilterTimeConstant=0.001  UdotUserProvided=0
  Simulink-PS Converter4 : nesl_utility/Simulink-PS Converter  Commented=on  PhysicalDomain=network_engine_domain  SubClassName=ps_input  LeftPortType=input  RightPortType=output  PseudoPeriodic=off  Frequencies=[]  NoiseDistribution=none  NoiseParameters=[]  Unit=1  AffineConversion=off  FilteringAndDerivatives=filter  SimscapeFilterOrder=2  InputFilterTimeConstant=0.001  UdotUserProvided=0
  Simulink-PS Converter5 : nesl_utility/Simulink-PS Converter  Commented=on  PhysicalDomain=network_engine_domain  SubClassName=ps_input  LeftPortType=input  RightPortType=output  PseudoPeriodic=off  Frequencies=[]  NoiseDistribution=none  NoiseParameters=[]  Unit=1  AffineConversion=off  FilteringAndDerivatives=filter  SimscapeFilterOrder=2  InputFilterTimeConstant=0.001  UdotUserProvided=0
  Simulink-PS Converter6 : nesl_utility/Simulink-PS Converter  Commented=on  PhysicalDomain=network_engine_domain  SubClassName=ps_input  LeftPortType=input  RightPortType=output  PseudoPeriodic=off  Frequencies=[]  NoiseDistribution=none  NoiseParameters=[]  Unit=1  AffineConversion=off  FilteringAndDerivatives=provide  SimscapeFilterOrder=1  InputFilterTimeConstant=0.001  UdotUserProvided=0
  Simulink-PS Converter7 : nesl_utility/Simulink-PS Converter  Commented=on  PhysicalDomain=network_engine_domain  SubClassName=ps_input  LeftPortType=input  RightPortType=output  PseudoPeriodic=off  Frequencies=[]  NoiseDistribution=none  NoiseParameters=[]  Unit=1  AffineConversion=off  FilteringAndDerivatives=provide  SimscapeFilterOrder=2  InputFilterTimeConstant=0.001  UdotUserProvided=0
  Simulink-PS Converter8 : nesl_utility/Simulink-PS Converter  Commented=on  PhysicalDomain=network_engine_domain  SubClassName=ps_input  LeftPortType=input  RightPortType=output  PseudoPeriodic=off  Frequencies=[]  NoiseDistribution=none  NoiseParameters=[]  Unit=1  AffineConversion=off  FilteringAndDerivatives=provide  SimscapeFilterOrder=1  InputFilterTimeConstant=0.001  UdotUserProvided=0
  Solver Configuration : nesl_utility/Solver Configuration  PhysicalDomain=network_engine_domain  SubClassName=solver  LeftPortType=input  RightPortType=generic  Tones=[]  Harmonics=[]  SimulateNoise=off  Profile=off  UseLocalSampling=off  EnableSwitchedLinearOptims=on  FrequencyDomain=off  UseCCode=off  RelTol=0.001  AbsTol=1e-06  MinStep=1e-09  ToWorkspace=off  RevertToSquareIcSolve=off  NumHomotopyIterations=100  PhasorMode=off  PhasorModeNumHarmonics=1  ConsistencySolver=NEWTON_FTOL  IndexReductionMethod=DerivativeReplacement  DoDC=off  ResidualTolerance=1e-09  ConsistencyTolSource=GLOBAL  ConsistencyAbsTol=0.001  ConsistencyRelTol=0.001  ConsistencyTolFactor=0.001  UseLocalSolver=off  LocalSolverChoice=NE_BACKWARD_EULER_ADVANCER  ResolveIndetEquations=on  FunctionEvalNumThread=1  LocalSolverSampleTime=0.001  DoFixedCost=off  MaxNonlinIter=3  MaxModeIter=2  ComputeImpulses=off  ImpulseIterations=2  LinearAlgebra=Sparse  LinearAlgebraNumThread=0  EquationFormulation=NE_TIME_EF  DelaysMemoryBudget=1024  AutomaticFiltering=on  FilteringTimeConstant=0.001  PartitionStorageMethod=AS_NEEDED  PartitionMemoryBudget=1024  PartitionMethod=FAST  MultibodyUseLocalSolver=off  MultibodyLocalSolverChoice=ODE1  MultibodyLocalSolverSampleTime=0.001
  Starship Rocket : sm_lib/Body Elements/File Solid  Commented=on  ExtGeomFileName=modell_raket.stl  UnitType=Custom  ExtGeomFileUnits=mm  StepReaderType=HEX  ExportConvexHullGeometry=off  InertiaType=CalculateFromGeometry  BasedOnType=Mass  Density=1000  DensityUnits=kg/m^3  Mass=3  MassUnits=kg  CenterOfMass=[66 38 534]  CenterOfMassUnits=mm  MomentsOfInertia=[1 1 1]  MomentsOfInertiaUnits=kg*m^2  ProductsOfInertia=[0 0 0]  ProductsOfInertiaUnits=kg*m^2  GraphicType=FromGeometry  MarkerShape=Sphere  MarkerSize=10  GraphicVisPropType=SimpleVisualProperties  GraphicDiffuseColor=[1.0 0.4 0.0]  GraphicOpacity=1.0  GraphicSpecularColor=[0.5 0.5 0.5 1.0]  GraphicAmbientColor=[0.15 0.15 0.15 1.0]  GraphicEmissiveColor=[0.0 0.0 0.0 1.0]  GraphicShininess=75  DoExposeReferenceFrame=on  SerializedFrames=<Frames><Frame><Id>Frame2</Id><Value><Name>Motor1</Name><Origin><Source>ReferenceFrame</Source><FeatureName></FeatureName></Origin><PrimaryAxis><DefinedDirection>+Z</DefinedDirection><Source>ReferenceFrame</Source><SourceDirection>+Z</SourceDirection><FeatureName></FeatureName></PrimaryAxis><SecondaryAxis><DefinedDirection>+X</DefinedDirection><Source>ReferenceFrame</Source><SourceDirection>+X</SourceDirection><FeatureName></FeatureName></SecondaryAxis></Value></Frame></Frames>
  "Translational acceleration " : Mux  Inputs=3
  Translational position : Mux  Inputs=3
  "Translational velocity " : Mux  Inputs=3
  Velocity : Scope
  Velocity x : nesl_utility/PS-Simulink Converter  PhysicalDomain=network_engine_domain  SubClassName=ps_output  LeftPortType=input  RightPortType=output  PseudoPeriodic=off  Frequencies=[]  VectorFormat=1-D array  Unit=inherit  AffineConversion=off
  Velocity y : nesl_utility/PS-Simulink Converter  PhysicalDomain=network_engine_domain  SubClassName=ps_output  LeftPortType=input  RightPortType=output  PseudoPeriodic=off  Frequencies=[]  VectorFormat=1-D array  Unit=inherit  AffineConversion=off
  Velocity z : nesl_utility/PS-Simulink Converter  PhysicalDomain=network_engine_domain  SubClassName=ps_output  LeftPortType=input  RightPortType=output  PseudoPeriodic=off  Frequencies=[]  VectorFormat=1-D array  Unit=inherit  AffineConversion=off
  Visual : sm_lib/Body Elements/File Solid  ExtGeomFileName=modell_raket.stl  UnitType=Custom  ExtGeomFileUnits=mm  StepReaderType=HEX  ExportConvexHullGeometry=off  InertiaType=Custom  BasedOnType=DensityFromFile  Density=1000  DensityUnits=kg/m^3  Mass=0  MassUnits=kg  CenterOfMass=[0 0 0]  CenterOfMassUnits=m  MomentsOfInertia=[0 0 0]  MomentsOfInertiaUnits=kg*m^2  ProductsOfInertia=[0 0 0]  ProductsOfInertiaUnits=kg*m^2  GraphicType=FromGeometry  MarkerShape=Sphere  MarkerSize=10  GraphicVisPropType=SimpleVisualProperties  GraphicDiffuseColor=[1.0 0.4 0.0]  GraphicOpacity=1.0  GraphicSpecularColor=[0.5 0.5 0.5 1.0]  GraphicAmbientColor=[0.15 0.15 0.15 1.0]  GraphicEmissiveColor=[0.0 0.0 0.0 1.0]  GraphicShininess=75  DoExposeReferenceFrame=on  SerializedFrames=<Frames/>
  World Frame : sm_lib/Frames and Transforms/World Frame
  h_1 : sm_lib/Frames and Transforms/Rigid Transform  RotationMethod=None  FollAlignAxisA=+X  BaseAlignAxisA=+Y  FollAlignAxisB=+Y  BaseAlignAxisB=+Z  RotationStandardAxis=+Z  RotationAngle=0  RotationAngleUnits=deg  RotationArbitraryAxis=[0 0 1]  RotationSequenceAxes=FollowerAxes  RotationSequence=XYX  RotationSequenceAngles=[0 0 0]  RotationSequenceAnglesUnits=deg  RotationMatrix=[1 0 0;0 1 0;0 0 1]  Quaternion=[1 0 0 0]  TranslationMethod=Cartesian  TranslationCartesianOffset=[0 0 -422]  TranslationCartesianOffsetUnits=mm  TranslationStandardAxis=+Z  TranslationStandardOffset=0  TranslationStandardOffsetUnits=m  TranslationROffset=0  TranslationROffsetUnits=m  TranslationThetaOffset=0  TranslationThetaOffsetUnits=deg  TranslationZOffset=0  TranslationZOffsetUnits=m
  h_2 : sm_lib/Frames and Transforms/Rigid Transform  RotationMethod=None  FollAlignAxisA=+X  BaseAlignAxisA=+Y  FollAlignAxisB=+Y  BaseAlignAxisB=+Z  RotationStandardAxis=+Z  RotationAngle=0  RotationAngleUnits=deg  RotationArbitraryAxis=[0 0 1]  RotationSequenceAxes=FollowerAxes  RotationSequence=XYX  RotationSequenceAngles=[0 0 0]  RotationSequenceAnglesUnits=deg  RotationMatrix=[1 0 0;0 1 0;0 0 1]  Quaternion=[1 0 0 0]  TranslationMethod=Cartesian  TranslationCartesianOffset=[0 0 -297]  TranslationCartesianOffsetUnits=mm  TranslationStandardAxis=+Z  TranslationStandardOffset=0  TranslationStandardOffsetUnits=m  TranslationROffset=0  TranslationROffsetUnits=m  TranslationThetaOffset=0  TranslationThetaOffsetUnits=deg  TranslationZOffset=0  TranslationZOffsetUnits=m
  kraft x : Step  Commented=on  Time=0  After=0  SampleTime=0
  kraft y : Step  Commented=on  Time=0  SampleTime=0
  noll : Step  Commented=on  Time=0  After=0  SampleTime=0
  x yaw acceleration : nesl_utility/PS-Simulink Converter  PhysicalDomain=network_engine_domain  SubClassName=ps_output  LeftPortType=input  RightPortType=output  PseudoPeriodic=off  Frequencies=[]  VectorFormat=1-D array  Unit=inherit  AffineConversion=off
  x yaw velocity : nesl_utility/PS-Simulink Converter  PhysicalDomain=network_engine_domain  SubClassName=ps_output  LeftPortType=input  RightPortType=output  PseudoPeriodic=off  Frequencies=[]  VectorFormat=1-D array  Unit=inherit  AffineConversion=off
  y pitch acceleration : nesl_utility/PS-Simulink Converter  PhysicalDomain=network_engine_domain  SubClassName=ps_output  LeftPortType=input  RightPortType=output  PseudoPeriodic=off  Frequencies=[]  VectorFormat=1-D array  Unit=inherit  AffineConversion=off
  y pitch velocity : nesl_utility/PS-Simulink Converter  PhysicalDomain=network_engine_domain  SubClassName=ps_output  LeftPortType=input  RightPortType=output  PseudoPeriodic=off  Frequencies=[]  VectorFormat=1-D array  Unit=inherit  AffineConversion=off
  z roll acceleration : nesl_utility/PS-Simulink Converter  PhysicalDomain=network_engine_domain  SubClassName=ps_output  LeftPortType=input  RightPortType=output  PseudoPeriodic=off  Frequencies=[]  VectorFormat=1-D array  Unit=inherit  AffineConversion=off
  z roll velocity : nesl_utility/PS-Simulink Converter  PhysicalDomain=network_engine_domain  SubClassName=ps_output  LeftPortType=input  RightPortType=output  PseudoPeriodic=off  Frequencies=[]  VectorFormat=1-D array  Unit=inherit  AffineConversion=off
  zero : Step  Commented=on  Time=0  After=0  SampleTime=0
  Px : Outport
  Pz : Outport  Port=2
  Py : Outport  Port=3
  Vx : Outport  Port=4
  Vy : Outport  Port=5
  Vz : Outport  Port=6
  gamma_1 : Outport  Port=7
  gamma_2 : Outport  Port=8
  gamma_1' : Outport  Port=9
  gamma_2' : Outport  Port=10
  wires:
  Position x/1 -> Camera/1(In1), Translational position/1, Px/1
  Velocity x/1 -> "Translational velocity "/1, Vx/1
  PS-Simulink Converter6/1 -> Quaternions to Rotation Angles/1
  x yaw velocity/1 -> gamma_2'/1, Angular vel./1
  y pitch velocity/1 -> Angular vel./2, gamma_1'/1
  Demux/1 -> gamma_2/1, Angular pos./1  "x yaw"
  Demux/2 -> Angular pos./2, gamma_1/1  "y pitch"
  Demux/3 -> Angular pos./3  "z roll"
  z roll velocity/1 -> Angular vel./3
  Constant/1 -> Simulink-PS Converter7/1
  Position y/1 -> Translational position/2, Camera/2(In2), Py/1
  Velocity y/1 -> Vy/1, "Translational velocity "/2
  Position z/1 -> Camera/3(In3), Translational position/3, Pz/1
  Velocity z/1 -> "Translational velocity "/3, Vz/1
  Translational position/1 -> Position/1
  "Translational velocity "/1 -> Velocity/1
  Angular vel./1 -> Angular velocity/1
  Acceleration x/1 -> "Translational acceleration "/1
  Acceleration y/1 -> "Translational acceleration "/2
  Acceleration z/1 -> "Translational acceleration "/3
  "Translational acceleration "/1 -> Acceleration/1
  Angular acc./1 -> Angular acceleration/1
  x yaw acceleration/1 -> Angular acc./1
  y pitch acceleration/1 -> Angular acc./2
  z roll acceleration/1 -> Angular acc./3
  Angular pos./1 -> Angular position/1
  F_1_z/1 -> Simulink-PS Converter2/1
  F_1_x/1 -> Simulink-PS Converter3/1
  F_2_z/1 -> Simulink-PS Converter1/1
  F_2_y/1 -> Simulink-PS Converter/1
  Quaternions to Rotation Angles/1 -> Demux/1
  noll/1 -> Simulink-PS Converter8/1
  kraft y/1 -> F_y/1
  kraft x/1 -> F_x/1
  zero/1 -> Simulink-PS Converter6/1
  connections:
  Position x/LConn1 -- 6-DOF Joint/RConn2
  World Frame/RConn1 -- Mechanism Configuration/RConn1 -- 6-DOF Joint/LConn1 -- Floor/LConn1 -- Camera/LConn1 -- Solver Configuration/RConn1
  Velocity x/LConn1 -- 6-DOF Joint/RConn3
  6-DOF Joint/RConn1 -- Rigid Transform/LConn1 -- Rocket/RConn1
  h_1/LConn1 -- Rocket/LConn2
  h_2/LConn1 -- Rocket/LConn1
  Simulink-PS Converter5/RConn1 -- Gimbal Joint/LConn2
  Simulink-PS Converter7/RConn1 -- Gimbal Joint/LConn3
  Simulink-PS Converter4/RConn1 -- Gimbal Joint1/LConn3
  6-DOF Joint/RConn5 -- Position y/LConn1
  6-DOF Joint/RConn6 -- Velocity y/LConn1
  6-DOF Joint/RConn8 -- Position z/LConn1
  6-DOF Joint/RConn9 -- Velocity z/LConn1
  6-DOF Joint/RConn11 -- PS-Simulink Converter6/LConn1
  6-DOF Joint/RConn12 -- x yaw velocity/LConn1
  6-DOF Joint/RConn13 -- y pitch velocity/LConn1
  6-DOF Joint/RConn14 -- z roll velocity/LConn1
  6-DOF Joint/RConn7 -- Acceleration y/LConn1
  6-DOF Joint/RConn10 -- Acceleration z/LConn1
  6-DOF Joint/RConn4 -- Acceleration x/LConn1
  6-DOF Joint/RConn17 -- z roll acceleration/LConn1
  y pitch acceleration/LConn1 -- 6-DOF Joint/RConn16
  6-DOF Joint/RConn15 -- x yaw acceleration/LConn1
  Force 2/RConn1 -- h_2/RConn1
  Force 1/RConn1 -- h_1/RConn1
  Rigid Transform/RConn1 -- Visual/RConn1
  Simulink-PS Converter/RConn1 -- Force 2/LConn1
  Simulink-PS Converter1/RConn1 -- Force 2/LConn2
  Simulink-PS Converter3/RConn1 -- Force 1/LConn1
  Simulink-PS Converter2/RConn1 -- Force 1/LConn2

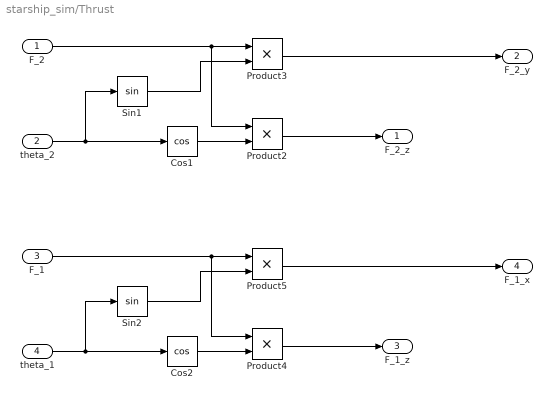
== system starship_sim/Thrust ==
  F_2 : Inport
  theta_2 : Inport  Port=2
  F_1 : Inport  Port=3
  theta_1 : Inport  Port=4
  Cos1 : Trigonometry  Operator=cos
  Cos2 : Trigonometry  Operator=cos
  Product{2..5} (4 alike) : Product  RndMeth=Zero
  Sin1 : Trigonometry
  Sin2 : Trigonometry
  F_2_z : Outport
  F_2_y : Outport  Port=2
  F_1_z : Outport  Port=3
  F_1_x : Outport  Port=4
  wires:
  Product3/1 -> F_2_y/1
  Cos1/1 -> Product2/2
  Sin1/1 -> Product3/2
  Product2/1 -> F_2_z/1
  theta_2/1 -> Cos1/1, Sin1/1
  F_2/1 -> Product2/1, Product3/1
  Sin2/1 -> Product5/2
  F_1/1 -> Product4/1, Product5/1
  Product5/1 -> F_1_x/1
  Product4/1 -> F_1_z/1
  Cos2/1 -> Product4/2
  theta_1/1 -> Cos2/1, Sin2/1

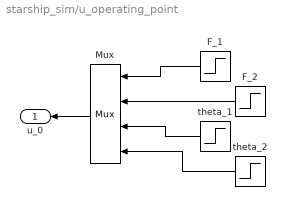
== system starship_sim/u_operating_point ==
  F_1 : Step  Time=0  After=13.74  SampleTime=0
  F_2 : Step  Time=0  After=13.74  SampleTime=0
  Mux : Mux
  theta_1 : Step  Time=0  After=0  SampleTime=0
  theta_2 : Step  Time=0  After=0  SampleTime=0
  u_0 : Outport
  wires:
  F_1/1 -> Mux/1
  F_2/1 -> Mux/2
  theta_2/1 -> Mux/4
  theta_1/1 -> Mux/3
  Mux/1 -> u_0/1

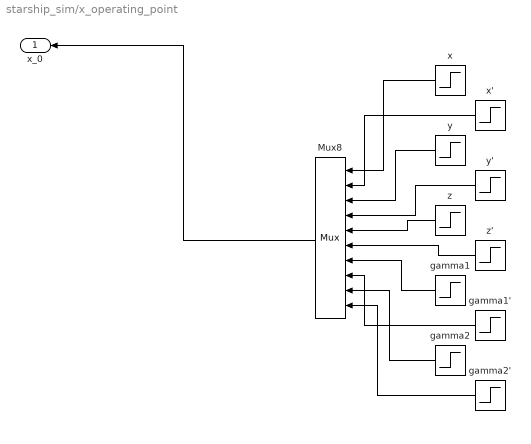
== system starship_sim/x_operating_point ==
  Mux8 : Mux  Inputs=10
  gamma1 : Step  Time=0  After=0  SampleTime=0
  gamma1' : Step  Time=0  After=0  SampleTime=0
  gamma2 : Step  Time=0  After=0  SampleTime=0
  gamma2' : Step  Time=0  After=0  SampleTime=0
  x : Step  Time=0  After=0  SampleTime=0
  x' : Step  Time=0  After=0  SampleTime=0
  y : Step  Time=0  After=0  SampleTime=0
  y' : Step  Time=0  After=0  SampleTime=0
  z : Step  Time=0  After=2  SampleTime=0
  z' : Step  Time=0  After=0  SampleTime=0
  x_0 : Outport
  wires:
  gamma1/1 -> Mux8/7
  gamma2/1 -> Mux8/9
  gamma1'/1 -> Mux8/8
  x'/1 -> Mux8/2
  y/1 -> Mux8/3
  x/1 -> Mux8/1
  gamma2'/1 -> Mux8/10
  y'/1 -> Mux8/4
  z/1 -> Mux8/5
  z'/1 -> Mux8/6
  Mux8/1 -> x_0/1
